simulink library "Power_Shaft1_Electric_A1"  (R2022a)
settings: Solver=VariableStepAuto  StartTime=0.0  StopTime=10.0  RelTol=1e-3
undefined symbols (not defined in the file): Powertrain
libraries: fl_lib x2, Power_Components x2, sm_lib x1, Cooling_Motor1_A1 x1
Description:
  | Component of Simscape Vehicle Templates Library
  | 
  | Copyright 2018-2024 The MathWorks, Inc.
settings Model: Creator=smiller  LastModifiedBy=smiller
settings SolverCC: AlgebraicLoopSolver=TrustRegion
settings DataIOCC: ReturnWorkspaceOutputs=off
settings DebuggingCC: UnconnectedInputMsg=warning  UnconnectedOutputMsg=warning  UnconnectedLineMsg=warning  SFMachineParentedDataDiag=warning  ArithmeticOperatorsInVariantConditions=warning
settings SFSimCC: CustomCodeUndefinedFunction=UseInterfaceOnly
settings RTWCC: DLArmComputeVersion=19.05

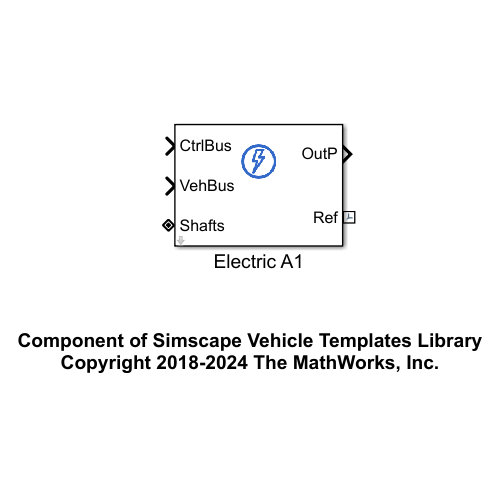
[thumbnail: Simulink's stored preview of the top-level diagram]
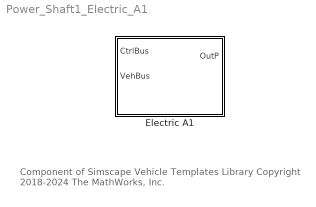
== system Power_Shaft1_Electric_A1 ==
  note: Component of Simscape Vehicle Templates Library
      | Copyright 2018-2024 The MathWorks, Inc.
  Electric A1 : Subsystem  VariantControl=ElectricTwoMotor  mask(Electric Propulsion with One Motor (FWD)){Power=Powertrain.Power}
      mask prompts: Power "Power1 Motor (Structure)"
      mask help: One electric motor with optional cooling system. Physical connection for the motor shaft are in bus Shafts and connect to a differential that powers the front axle.
      mask Display: image('sm_car_vehicle_power_e1motor_A1_IMAGE.png');

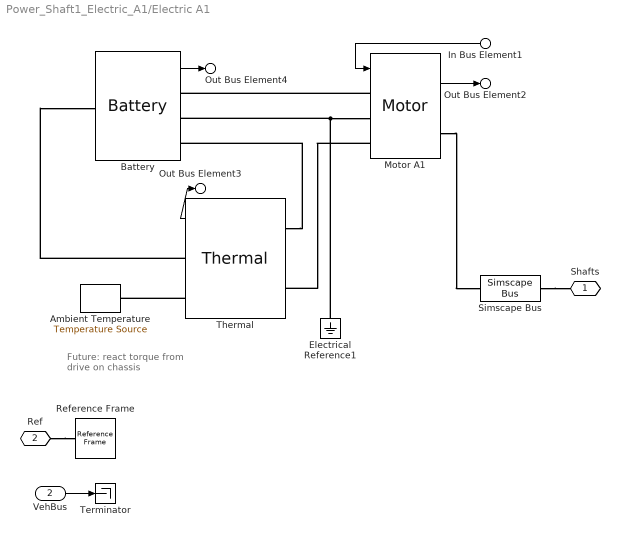
== system Power_Shaft1_Electric_A1/Electric A1 ==
  note: Future:
      | react torque
      | from drive
      | on chassis
  In Bus Element1 : Inport  PortName=CtrlBus  Element=MMotorA1Demand
  VehBus : Inport  Port=2
  Ambient Temperature : fl_lib/Thermal/Thermal Sources/Temperature Source  temperature=Power.TAmbient.Value K
      settings: SourceProductBaseCode=PW,SS,VE
  Battery : Power_Components/Battery  SystemSampleTime=-1  VariantActivationTime=update diagram  Latency=0  AutoFrameSizeCalculation=off
  Electrical Reference1 : fl_lib/Electrical/Electrical Elements/Electrical Reference
      settings: SourceProductBaseCode=PW,SS,VE
  Motor A1 : Power_Components/Motor  Motor=Power.MotorA1
  Reference Frame : sm_lib/Frames and Transforms/Reference Frame
  Simscape Bus : SimscapeBus  HierarchyStrings=ShaftA1
  Terminator : Terminator
  Thermal : Cooling_Motor1_A1/Thermal  VariantControl=Variant1  LabelModeActiveChoice=Liquid_Loop1  VariantLabel=Power.Cooling.class.Value
      settings: AttributesFormatString=%<ActiveVariant>
  Shafts : PMIOPort  Side=Left
  Ref : PMIOPort  Port=2  Side=Right
  Out Bus Element2 : Outport  VectorParamsAs1DForOutWhenUnconnected=off  PortName=OutP  Element=MotorA1
  Out Bus Element3 : Outport  VectorParamsAs1DForOutWhenUnconnected=off  PortName=OutP  Element=Thermal
  Out Bus Element4 : Outport  VectorParamsAs1DForOutWhenUnconnected=off  PortName=OutP  Element=Battery
  wires:
  In Bus Element1/1 -> Motor A1/1
  Motor A1/1 -> Out Bus Element2/1
  Thermal/1 -> Out Bus Element3/1
  VehBus/1 -> Terminator/1
  Battery/1 -> Out Bus Element4/1
  connections:
  Motor A1/LConn1 -- Battery/RConn1
  Electrical Reference1/LConn1 -- Battery/RConn2 -- Motor A1/LConn2
  Motor A1/RConn1 -- Simscape Bus/LConn1
  Simscape Bus/RConn1 -- Shafts/RConn1
  Ref/RConn1 -- Reference Frame/RConn1
  Thermal/LConn1 -- Battery/RConn3
  Motor A1/LConn3 -- Thermal/LConn2
  Thermal/RConn2 -- Ambient Temperature/LConn1
  Thermal/RConn1 -- Battery/LConn1
